simulink library "ITKLib"  (R2022b)
settings: Solver=FixedStepDiscrete  StartTime=0.0  StopTime=10.0  FixedStep=0.01  RelTol=1e-3  EnableMultiTasking=on
values from neighbouring files (symbols this model uses):
  Glb_WhlRollgRd_SC = single(0.36)    [init_Global.m]
undefined symbols (not defined in the file or in its folder): docblock, SlDemoSign, SlDemoSign_Positive_SC, TaskTime_100ms_SC, TaskTime_10ms_SC, VehRefSpd_vMaxRefSpd_C
libraries: simulink x51, $bdroot x45, ITKLib_V14 x1
(part 9 of 10)

== system ITKLib/TimeCounter/CounterRStep ==
  E : Inport  OutDataTypeStr=boolean
  R : Inport  Port=2  OutDataTypeStr=boolean
  Inc : Inport  Port=3
  Constant3 : Constant  Value=Cnt_Max  OutDataTypeStr=uint16  SampleTime=-1
  Limit : Subsystem  Description=""  mask(LIMIT_SL){}
      mask help:
      | GAC Library for Function Development
      |
      | Limits the input value u between the maximum (MX) and the minimum (MN) values.
      |
      | The input value u is checked first against the minimum value and then against the maximum value.
      |
      | In addition to that a flag is set in case the current value is higher than MX and another flag is set in case the current value is smaller than the MN value.
      |
      | inputs:
      | MX  - maximum allowed value
      | MN  - minimal allowed value
      | u   - input value to be evaluated
      |
      | outputs:
      | y       - limited output value
      mask Display:
      | color('black');
      | plot([0.2,0.8],[0.5,0.5]);
      | plot([0.5,0.5],[0.2,0.8]);
      | plot([0.75,0.8,0.75],[0.53,0.5,0.47]);
      | plot([0.53,0.5,0.47],[0.75,0.8,0.75]);
      | color('blue');
      | plot([0.2,0.3,0.7,0.8],[0.3,0.3,0.7,0.7]);
  Limit1 : Subsystem  Description=""  mask(LimitWoFlag){}
      mask help:
      | Limits the input value u between the maximum (MX) and the minimum (MN) values.
      |
      | The input value u is checked first against the minimum value and then against the maximum value.
      |
      | In addition to that a flag is set in case the current value is higher than MX and another flag is set in case the current value is smaller than the MN value.
      |
      | inputs:
      | MX  - maximum allowed value
      | MN  - minimal allowed value
      | u   - input value to be evaluated
      |
      | outputs:
      | y       - limited output value
      |
      | Simulink Custom Model Library, created by MCC.
      mask Display:
      | color('black');
      | plot([0.2,0.8],[0.5,0.5]);
      | plot([0.5,0.5],[0.2,0.8]);
      | plot([0.75,0.8,0.75],[0.53,0.5,0.47]);
      | plot([0.53,0.5,0.47],[0.75,0.8,0.75]);
      | color('blue');
      | plot([0.2,0.3,0.7,0.8],[0.3,0.3,0.7,0.7]);
  Number1 : Constant  Value=65535  OutDataTypeStr=uint16
      settings: AttributesFormatString=%<OutDataTypeStr>
  Number2 : Constant  Value=0  OutDataTypeStr=uint16
      settings: AttributesFormatString=%<OutDataTypeStr>
  Number3 : Constant  Value=0  OutDataTypeStr=uint16
      settings: AttributesFormatString=%<OutDataTypeStr>
  Number8 : Constant  Value=0  OutDataTypeStr=uint16
      settings: AttributesFormatString=%<OutDataTypeStr>
  Saturation2 : Saturate  UpperLimit=uint16(65534)  LowerLimit=uint16(0)
      settings: AttributesFormatString=|
      | UpperLimit = %<UpperLimit>
      | LowLimit = %<LowerLimit>
  Sum : Sum  InputSameDT=on  OutDataTypeStr=uint16  SaturateOnIntegerOverflow=on
  Switch1 : Switch  Criteria=u2 ~= 0  OutDataTypeStr=uint16
      settings: AttributesFormatString=threshold=%<threshold>\nCriteria : %<Criteria>
  Switch2 : Switch  Criteria=u2 ~= 0
      settings: AttributesFormatString=threshold=%<threshold>\nCriteria : %<Criteria>
  Unit Delay1 : UnitDelay  InitialCondition=uint16(0)  SampleTime=-1  HasFrameUpgradeWarning=on
      settings: AttributesFormatString=<initial=%<x0>>
  Cnt : Outport
  wires:
  E/1 -> Switch1/2
  Unit Delay1/1 -> Sum/2, Switch1/3
  Number2/1 -> Switch2/1
  Sum/1 -> Saturation2/1
  Switch1/1 -> Switch2/3
  Inc/1 -> Limit/2(u)
  R/1 -> Switch2/2
  Limit1/1(y) -> Cnt/1, Unit Delay1/1
  Switch2/1 -> Limit1/2(u)
  Constant3/1 -> Limit1/1(MX)
  Number3/1 -> Limit1/3(MN)
  Limit/1(y) -> Sum/1
  Number1/1 -> Limit/1(MX)
  Number8/1 -> Limit/3(MN)
  Saturation2/1 -> Switch1/1

== system ITKLib/TimeCounter/DebCnt ==
  bErr : Inport  OutDataTypeStr=boolean
  bRst : Inport  Port=2  OutDataTypeStr=boolean
  bEna : Inport  Port=3  OutDataTypeStr=boolean  PortDimensions=1
  FailThd : Inport  Port=4  OutDataTypeStr=int16
  RcvThd : Inport  Port=5  OutDataTypeStr=int16
  IncFail : Inport  Port=6  OutDataTypeStr=int16
  DecRcv : Inport  Port=7  OutDataTypeStr=int16
  DebounceEnable : Subsystem
  Debounce_OBD : Subsystem  TreatAsAtomicUnit=on
  Unit Delay1 : UnitDelay  SampleTime=-1  HasFrameUpgradeWarning=on
      settings: AttributesFormatString=<initial=%<X0>>
  Unit Delay2 : UnitDelay  SampleTime=-1  HasFrameUpgradeWarning=on
      settings: AttributesFormatString=<initial=%<X0>>
  bFaild : Outport
  wires:
  DecRcv/1 -> Debounce_OBD/6(DecrRec)
  IncFail/1 -> Debounce_OBD/5(IncrFail)
  Debounce_OBD/2(bFaild) -> Unit Delay1/1, bFaild/1
  bErr/1 -> DebounceEnable/5(bErr), Debounce_OBD/1(bErr)
  bRst/1 -> Debounce_OBD/2(bRst), DebounceEnable/4(bRst)
  FailThd/1 -> Debounce_OBD/3(FailThd)
  RcvThd/1 -> Debounce_OBD/4(RecThd)
  bEna/1 -> DebounceEnable/3(bEna)
  Debounce_OBD/1(bOutRanged) -> Unit Delay2/1
  DebounceEnable/1(bDebounceEna) -> Debounce_OBD/Enable
  Unit Delay2/1 -> DebounceEnable/1(bOutRangedOld)
  Unit Delay1/1 -> DebounceEnable/2(bFailedOld)

== system ITKLib/TimeCounter/Debounce ==
  In : Inport  OutDataTypeStr=boolean
  R : Inport  Port=2
  TAct : Inport  Port=3
  TDeact : Inport  Port=4
  dT : Inport  Port=5
  Constant2 : Constant  Value=IV  OutDataTypeStr=boolean  SampleTime=-1
  Logical Operator1 : Logic  Operator=NOT  AllPortsSameDT=off  OutDataTypeStr=boolean
  OR : Logic  Operator=OR  OutDataTypeStr=boolean
  RSLatchIV : Subsystem  RTWFcnName=RS_Latch_IV_Pos  RTWFileName=SEN_MDL_LIB  mask(RSLatchIV){}
      mask help:
      | RS latch with initial value
      | Set signal is passed from port 'S'
      | Reset signal is passed from port 'R'
      | Initial value is passed from port 'IV'
      |
      | Q is set if S is set and reset if R is set.
      | The reset logic is of higher priority than set logic.
      | The initial state is set by IV.
      |
      | Simulink Custom Model Library, created by MCC.
      settings: MinAlgLoopOccurrences=on  RTWFcnNameOpts=User specified  RTWFileNameOpts=User specified
      mask Help:
      | RS latch with initial value
      | Set signal is passed from port 'S'
      | Reset signal is passed from port 'R'
      | Initial value is passed from port 'IV'
      | 
      | Q is set if S is set and reset if R is set.
      | The reset logic is of higher priority than set logic.
      | The initial state is set by IV.
      mask Display:
      | color('blue')
      | disp('\fontsize{12}RS Latch', 'texmode', 'on')
      | color('black');
      | port_label('input', 1, 'S', 'texmode', 'on')
      | port_label('input', 2, 'R', 'texmode', 'on')
      | port_label('input', 3, 'IV', 'texmode', 'on')
      | port_label('output', 1, 'Q', 'texmode', 'on')
      | %text(1,0,'SEN','horizontalAlignment','right','verticalAlignment','bottom');
  TurnOnDelayVari : $bdroot/TimeCounter/TurnOnDelayVari
      settings: AttributesFormatString=TurnOnDelay
  TurnOnDelayVari1 : $bdroot/TimeCounter/TurnOnDelayVari
      settings: AttributesFormatString=TurnOnDelay
  Out : Outport  OutDataTypeStr=boolean
  wires:
  Constant2/1 -> RSLatchIV/3(IV)
  RSLatchIV/1(Q) -> Out/1
  TAct/1 -> TurnOnDelayVari/3
  dT/1 -> [dT], TurnOnDelayVari/2
  TDeact/1 -> TurnOnDelayVari1/3
  In/1 -> TurnOnDelayVari/1, Logical Operator1/1
  Logical Operator1/1 -> TurnOnDelayVari1/1
  TurnOnDelayVari/1 -> RSLatchIV/1(S)
  R/1 -> OR/2
  OR/1 -> RSLatchIV/2(R)
  TurnOnDelayVari1/1 -> OR/1
  [dT] -> TurnOnDelayVari1/2

== system ITKLib/TimeCounter/StopWatchRE ==
  E : Inport  OutDataTypeStr=boolean
  R : Inport  Port=2  OutDataTypeStr=boolean
  dT : Inport  Port=3
  Number1 : Constant  Value=0  OutDataTypeStr=single
      settings: AttributesFormatString=%<OutDataTypeStr>
  Sum1 : Sum  SaturateOnIntegerOverflow=on
  Switch1 : Switch  Criteria=u2 ~= 0  SaturateOnIntegerOverflow=off  InputSameDT=off
      settings: AttributesFormatString=Criteria : %<Criteria>
  Switch2 : Switch  Criteria=u2 ~= 0  SaturateOnIntegerOverflow=off  InputSameDT=off
      settings: AttributesFormatString=Criteria : %<Criteria>
  Unit Delay1 : UnitDelay  SampleTime=-1  HasFrameUpgradeWarning=on
      settings: AttributesFormatString=<initial=%<x0>>
  y : Outport
  wires:
  dT/1 -> Sum1/1
  Switch2/1 -> y/1, Unit Delay1/1
  Switch1/1 -> Switch2/3
  E/1 -> Switch1/2
  Number1/1 -> Switch2/1
  R/1 -> Switch2/2
  Unit Delay1/1 -> Switch1/3, Sum1/2
  Sum1/1 -> Switch1/1

== system ITKLib/TimeCounter/TurnOnDelayVari ==
  In : Inport  OutDataTypeStr=boolean
  dT : Inport  Port=2
  T : Inport  Port=3
  DataTypeConversion : DataTypeConversion  OutDataTypeStr=int32  RndMeth=Nearest  SaturateOnIntegerOverflow=off
  Divide : Product  Inputs=*/  InputSameDT=on  SaturateOnIntegerOverflow=on
  Max : MinMax  Function=max  Inputs=2  InputSameDT=on  SaturateOnIntegerOverflow=on
  Relational Operator1 : RelationalOperator  Operator=>  OutDataTypeStr=boolean
  Saturation2 : Saturate  UpperLimit=2147483647  LowerLimit=-2147483648
      settings: AttributesFormatString=|
      | UpperLimit = %<UpperLimit>
      | LowLimit = %<LowerLimit>
  Subtract1 : Sum  InputSameDT=on  SaturateOnIntegerOverflow=on
  Switch : Switch  Criteria=u2 ~= 0  SaturateOnIntegerOverflow=off  InputSameDT=off
      settings: AttributesFormatString=Criteria : %<Criteria>
  Unit Delay : UnitDelay  InitialCondition=int32(0)  SampleTime=-1  HasFrameUpgradeWarning=on
      settings: AttributesFormatString=<initial=%<x0>>
  single1 : Constant  OutDataTypeStr=int32
      settings: AttributesFormatString=%<OutDataTypeStr>
  single2 : Constant  Value=0  OutDataTypeStr=int32
      settings: AttributesFormatString=%<OutDataTypeStr>
  single3 : Constant  Value=0.0001  OutDataTypeStr=single
      settings: AttributesFormatString=%<OutDataTypeStr>
  Out : Outport  OutDataTypeStr=boolean
  wires:
  single2/1 -> Switch/3
  In/1 -> Switch/2
  Switch/1 -> Saturation2/1
  Relational Operator1/1 -> Out/1
  Subtract1/1 -> Switch/1
  Unit Delay/1 -> Subtract1/1
  single1/1 -> Subtract1/2
  Divide/1 -> DataTypeConversion/1
  DataTypeConversion/1 -> Relational Operator1/2
  T/1 -> Divide/1
  dT/1 -> Max/1
  single3/1 -> Max/2
  Max/1 -> Divide/2
  Saturation2/1 -> Unit Delay/1, Relational Operator1/1

== system ITKLib/TimeCounter/Turn_Off_Delay_Vari ==
  In : Inport  OutDataTypeStr=boolean
  dT : Inport  Port=2
  T : Inport  Port=3
  DataTypeConversion : DataTypeConversion  OutDataTypeStr=int32  RndMeth=Nearest  SaturateOnIntegerOverflow=off
  Divide : Product  Inputs=*/  InputSameDT=on  SaturateOnIntegerOverflow=on
  Logical Operator2 : Logic  Operator=OR  AllPortsSameDT=off  OutDataTypeStr=boolean
  Max : MinMax  Function=max  Inputs=2  InputSameDT=on  SaturateOnIntegerOverflow=on
  Relational Operator : RelationalOperator  Operator=>  OutDataTypeStr=boolean  InputSameDT=off
  Saturation2 : Saturate  UpperLimit=2147483647  LowerLimit=-2147483648
      settings: AttributesFormatString=|
      | UpperLimit = %<UpperLimit>
      | LowLimit = %<LowerLimit>
  Subtract : Sum  Inputs=+-
  Switch : Switch  Criteria=u2 ~= 0  SaturateOnIntegerOverflow=off  InputSameDT=off
      settings: AttributesFormatString=Criteria : %<Criteria>
  Switch1 : Switch  Criteria=u2 ~= 0  SaturateOnIntegerOverflow=off  InputSameDT=off
      settings: AttributesFormatString=Criteria : %<Criteria>
  Unit Delay : UnitDelay  InitialCondition=uint32(0)  SampleTime=-1  HasFrameUpgradeWarning=on
      settings: AttributesFormatString=<initial=%<x0>>
  single3 : Constant  Value=0.0001  OutDataTypeStr=single
      settings: AttributesFormatString=%<OutDataTypeStr>
  single4 : Constant  Value=0  OutDataTypeStr=int32
      settings: AttributesFormatString=%<OutDataTypeStr>
  single5 : Constant  OutDataTypeStr=int32
      settings: AttributesFormatString=%<OutDataTypeStr>
  Out : Outport  OutDataTypeStr=boolean
  wires:
  Switch/1 -> Saturation2/1
  single4/1 -> Relational Operator/2
  Logical Operator2/1 -> Out/1
  Switch1/1 -> Switch/3
  Relational Operator/1 -> Switch1/2, [TimeFlag]
  In/1 -> Switch/2, Logical Operator2/2
  Unit Delay/1 -> Subtract/1, Relational Operator/1, Switch1/3
  Subtract/1 -> Switch1/1
  [TimeFlag] -> Logical Operator2/1
  DataTypeConversion/1 -> Switch/1
  single5/1 -> Subtract/2
  Max/1 -> Divide/2
  single3/1 -> Max/2
  dT/1 -> Max/1
  T/1 -> Divide/1
  Divide/1 -> DataTypeConversion/1
  Saturation2/1 -> Unit Delay/1

== system ITKLib/BasicOperators/Drvt/MaxITK ==
  In1 : Inport
  In2 : Inport  Port=2
  Greater : RelationalOperator  Operator=>  OutDataTypeStr=boolean
  Switch : Switch  Criteria=u2 ~= 0  SaturateOnIntegerOverflow=off  InputSameDT=off
      settings: AttributesFormatString=Criteria : %<Criteria>
  Out1 : Outport  VectorParamsAs1DForOutWhenUnconnected=off
  wires:
  In1/1 -> Switch/1, Greater/1
  In2/1 -> Switch/3, Greater/2
  Greater/1 -> Switch/2
  Switch/1 -> Out1/1

== system ITKLib/BasicOperators/Int32ToSingle/Opposite ==
  In : Inport
  Product2 : Product  InputSameDT=on  SaturateOnIntegerOverflow=on
  single : Constant  Value=-1  OutDataTypeStr=single
      settings: AttributesFormatString=%<OutDataTypeStr>
  " Out " : Outport
  wires:
  single/1 -> Product2/2
  Product2/1 -> " Out "/1
  In/1 -> Product2/1

== system ITKLib/BasicOperators/Safe_Divide/Opposite ==
  In : Inport
  Product2 : Product  InputSameDT=on  SaturateOnIntegerOverflow=on
  single : Constant  Value=-1  OutDataTypeStr=single
      settings: AttributesFormatString=%<OutDataTypeStr>
  " Out " : Outport
  wires:
  single/1 -> Product2/2
  Product2/1 -> " Out "/1
  In/1 -> Product2/1

== system ITKLib/BasicOperators/Safe_Divide/Opposite1 ==
  In : Inport
  Product2 : Product  InputSameDT=on  SaturateOnIntegerOverflow=on
  single : Constant  Value=-1  OutDataTypeStr=single
      settings: AttributesFormatString=%<OutDataTypeStr>
  " Out " : Outport
  wires:
  single/1 -> Product2/2
  Product2/1 -> " Out "/1
  In/1 -> Product2/1

== system ITKLib/Diagnosis/Debounce_OBD/DebounceEnable ==
  bOutRangedOld : Inport
  bFailedOld : Inport  Port=2
  bEna : Inport  Port=3  OutDataTypeStr=boolean  PortDimensions=1
  bRst : Inport  Port=4
  bErr : Inport  Port=5
  Logical Operator : Logic  Operator=OR  OutDataTypeStr=boolean
  Logical Operator1 : Logic  OutDataTypeStr=boolean
  Logical Operator2 : Logic  Operator=NOT  Inputs=1  AllPortsSameDT=off  OutDataTypeStr=boolean
  Logical Operator3 : Logic  OutDataTypeStr=boolean
  Logical Operator4 : Logic  Inputs=1  AllPortsSameDT=off  OutDataTypeStr=boolean
  Relational Operator : RelationalOperator  Operator===  OutDataTypeStr=boolean
  bDebounceEna : Outport
  wires:
  bEna/1 -> Logical Operator3/2
  Logical Operator3/1 -> Logical Operator/1
  Logical Operator/1 -> bDebounceEna/1
  Relational Operator/1 -> Logical Operator1/2
  Logical Operator1/1 -> Logical Operator4/1
  Logical Operator2/1 -> Logical Operator3/1
  bOutRangedOld/1 -> Logical Operator1/1
  Logical Operator4/1 -> Logical Operator2/1
  bErr/1 -> Relational Operator/2
  bRst/1 -> Logical Operator/2
  bFailedOld/1 -> Relational Operator/1

== system ITKLib/Diagnosis/Debounce_OBD/Debounce_OBD ==
  note: test run failure always causes fault detection counter to increment above 0
      | (so as not to double the fail detection time following a test complete with pass)
  note: only if the FaultDetectionCounter less than 0
  note: rising edge detection
  note: FailCtr <= errCtr <= RecoverCtr
  bErr : Inport
  bRst : Inport  Port=2
  FailThd : Inport  Port=3
  RecThd : Inport  Port=4
  IncrFail : Inport  Port=5
  DecrRec : Inport  Port=6
  Enable : EnablePort
  EdgeRising : $bdroot/Memory/EdgeRising  Tag=initial value = 0
  LORelay1 : Logic  Operator=OR  AllPortsSameDT=off  OutDataTypeStr=boolean
  Logical Operator : Logic  OutDataTypeStr=boolean
  ROLoLim : RelationalOperator  Operator=<  OutDataTypeStr=boolean  InputSameDT=off
  ROUpLim : RelationalOperator  Operator=<  OutDataTypeStr=boolean  InputSameDT=off
  RSLatch : $bdroot/Memory/RSLatch
  Relational Operator : RelationalOperator  Operator=<  OutDataTypeStr=boolean
  Saturation2 : Saturate  UpperLimit=int16(32766)  LowerLimit=int16(-32767)
      settings: AttributesFormatString=|
      | UpperLimit = %<UpperLimit>
      | LowLimit = %<LowerLimit>
  Sum1 : Sum  InputSameDT=on  OutDataTypeStr=int16  SaturateOnIntegerOverflow=on
  Sum2 : Sum  InputSameDT=on  OutDataTypeStr=int16  SaturateOnIntegerOverflow=on
  Switch{,2..4} (4 alike) : Switch  Criteria=u2 ~= 0  SaturateOnIntegerOverflow=off  InputSameDT=off
      settings: AttributesFormatString=Criteria : %<Criteria>
  Unit Delay : UnitDelay  SampleTime=-1  HasFrameUpgradeWarning=on
      settings: AttributesFormatString=<initial=%<X0>>
  int1 : Constant  Value=0  OutDataTypeStr=int16
      settings: AttributesFormatString=%<OutDataTypeStr>
  int16 : Constant  Value=0  OutDataTypeStr=int16
      settings: AttributesFormatString=%<OutDataTypeStr>
  bOutRanged : Outport  InitialOutput=0
  bFailed : Outport  Port=2  InitialOutput=0
  wires:
  [bRst] -> Switch2/2
  Switch2/1 -> Switch3/1, Sum2/2, Sum1/2
  Switch/1 -> Switch2/3
  int16/1 -> Switch2/1, Switch/1
  RSLatch/1 -> bFailed/1
  Sum1/1 -> Switch4/1
  Sum2/1 -> Switch4/3
  Switch3/1 -> Unit Delay/1
  DecrRec/1 -> Sum2/1
  IncrFail/1 -> Sum1/1
  bErr/1 -> Switch4/2, EdgeRising/1
  Logical Operator/1 -> Switch/2
  Relational Operator/1 -> Logical Operator/2
  int1/1 -> Relational Operator/2
  EdgeRising/1 -> Logical Operator/1
  Unit Delay/1 -> Relational Operator/1, Switch/3
  bRst/1 -> [bRst], LORelay1/2
  RecThd/1 -> ROLoLim/2
  ROUpLim/1 -> RSLatch/1, Switch3/2, bOutRanged/1  "outRanged"
  Switch4/1 -> Saturation2/1
  ROLoLim/1 -> LORelay1/1
  FailThd/1 -> ROUpLim/1
  LORelay1/1 -> RSLatch/2
  Saturation2/1 -> Switch3/3, ROLoLim/1, ROUpLim/2

== system ITKLib/Diagnosis/FltCollctn/FltPos ==
  FltNr : Inport
  Divide : Product  Inputs=*/
  Math Function : Math  Operator=mod  SignedPower=on
  uint8 : Constant  Value=16  OutDataTypeStr=uint8  SampleTime=-1
      settings: AttributesFormatString=%<OutDataTypeStr>
  AryIdx : Outport
  BitPos : Outport  Port=2
  wires:
  Math Function/1 -> BitPos/1
  Divide/1 -> AryIdx/1
  FltNr/1 -> Divide/1, Math Function/1
  uint8/1 -> Math Function/2, Divide/2

== system ITKLib/Diagnosis/FltLatchCollctn/FltPos ==
  FltNr : Inport
  Divide : Product  Inputs=*/
  Math Function : Math  Operator=mod  SignedPower=on
  uint8 : Constant  Value=16  OutDataTypeStr=uint8  SampleTime=-1
      settings: AttributesFormatString=%<OutDataTypeStr>
  AryIdx : Outport
  BitPos : Outport  Port=2
  wires:
  uint8/1 -> Divide/2, Math Function/2
  FltNr/1 -> Math Function/1, Divide/1
  Divide/1 -> AryIdx/1
  Math Function/1 -> BitPos/1

== system ITKLib/Diagnosis/FltLatchCollctn/Subsystem ==
  FltNr : Inport
  FltFlg : Inport  Port=2
  SentCod : Inport  Port=3
  AND : Logic  OutDataTypeStr=boolean
  Demux : Demux
  Equal{,1..3} (4 alike) : RelationalOperator  Operator===  OutDataTypeStr=boolean  RndMeth=Simplest  InputSameDT=off
  Not : Logic  Operator=NOT  AllPortsSameDT=off  OutDataTypeStr=boolean
  OR : Logic  Operator=OR  Inputs=4  OutDataTypeStr=boolean
  RSLatch : $bdroot/Memory/RSLatch
  FltFlg1 : Outport
  wires:
  FltFlg/1 -> Not/1, RSLatch/1
  Demux/1 -> Equal/1
  Not/1 -> AND/2
  Demux/4 -> Equal3/1
  AND/1 -> RSLatch/2
  FltNr/1 -> Equal/2, Equal1/2, Equal2/2, Equal3/2
  Equal2/1 -> OR/3
  Demux/2 -> Equal1/1
  Equal3/1 -> OR/4
  Equal/1 -> OR/1
  OR/1 -> AND/1
  Equal1/1 -> OR/2
  Demux/3 -> Equal2/1
  RSLatch/1 -> FltFlg1/1
  SentCod/1 -> Demux/1

== system ITKLib/Diagnosis/RollgCntrChk/RSLatch ==
  S : Inport  OutDataTypeStr=boolean
  R : Inport  Port=2  OutDataTypeStr=boolean
  Logical Operator1 : Logic  Operator=NOT  AllPortsSameDT=off  OutDataTypeStr=boolean
  Logical_Operator4 : Logic  AllPortsSameDT=off  OutDataTypeStr=boolean
  Logical_Operator5 : Logic  Operator=OR  AllPortsSameDT=off  OutDataTypeStr=boolean
  Unit Delay : UnitDelay  SampleTime=-1  HasFrameUpgradeWarning=on
      settings: AttributesFormatString=<initial=%<x0>>
  Q : Outport  OutDataTypeStr=boolean
  wires:
  Unit Delay/1 -> Logical_Operator5/2
  Logical_Operator4/1 -> Q/1, Unit Delay/1
  Logical Operator1/1 -> Logical_Operator4/1
  Logical_Operator5/1 -> Logical_Operator4/2
  R/1 -> Logical Operator1/1
  S/1 -> Logical_Operator5/1

== system ITKLib/Filter/MoveAvrgFilt/Limit1 ==
  MX : Inport
  u : Inport  Port=2
  MN : Inport  Port=3
  GreaterOrEqual : RelationalOperator  OutDataTypeStr=boolean
  MinMax : MinMax  Inputs=2  SaturateOnIntegerOverflow=on
  MinMax1 : MinMax  Function=max  Inputs=2  SaturateOnIntegerOverflow=on
  MinMax2 : MinMax  Function=max  Inputs=2  SaturateOnIntegerOverflow=on
  MinMax3 : MinMax  Inputs=2  SaturateOnIntegerOverflow=on
  Switch : Switch  Criteria=u2 ~= 0  SaturateOnIntegerOverflow=off  InputSameDT=off
      settings: AttributesFormatString=Criteria : %<Criteria>
  y : Outport  InitialOutput=0
  wires:
  [MX] -> MinMax/1
  [MN] -> MinMax1/2
  MinMax3/1 -> Switch/3
  [MN] -> MinMax3/2
  MinMax2/1 -> MinMax3/1
  [MX] -> MinMax2/2
  [u] -> MinMax2/1
  MinMax/1 -> Switch/1
  GreaterOrEqual/1 -> Switch/2
  Switch/1 -> y/1
  MinMax1/1 -> MinMax/2
  MN/1 -> GreaterOrEqual/2, [MN]
  u/1 -> MinMax1/1, [u]
  MX/1 -> GreaterOrEqual/1, [MX]

== system ITKLib/Filter/SecOrdBPF/DisableFilterDeal ==
  Input : Inport
  ActionPort : ActionPort  InitializeStates=reset  ActionPortLabel=else
  Output : Outport
  wires:
  Input/1 -> Output/1

== system ITKLib/Filter/SecOrdBPF/FilterJudgment ==
  FilterTime : Inport
  SampleTime : Inport  Port=2
  LogicalOperator : Logic  AllPortsSameDT=off  OutDataTypeStr=boolean
  RelationalOperator : RelationalOperator  Operator=>  OutDataTypeStr=boolean  RndMeth=Simplest  InputSameDT=off
  RelationalOperator2 : RelationalOperator  Operator=>  OutDataTypeStr=boolean  RndMeth=Simplest  InputSameDT=off
  single4 : Constant  Value=0  OutDataTypeStr=single  SampleTime=-1
      settings: AttributesFormatString=%<OutDataTypeStr>
  u1 : Outport
  wires:
  LogicalOperator/1 -> u1/1
  RelationalOperator2/1 -> LogicalOperator/2
  single4/1 -> RelationalOperator2/2
  RelationalOperator/1 -> LogicalOperator/1
  SampleTime/1 -> RelationalOperator/2, RelationalOperator2/1
  FilterTime/1 -> RelationalOperator/1

== system ITKLib/Filter/SecOrdBPF/If Action Subsystem ==
  in : Inport
  FltOutOld : Inport  Port=2
  Omega : Inport  Port=3
  Zeta : Inport  Port=4
  SmpTime : Inport  Port=5
  Action Port : ActionPort  InitializeStates=reset  ActionPortLabel=if(u1 ~=0)
  Add : Sum  Inputs=+++
  Add1 : Sum  Inputs=+-+
  Add2 : Sum  Inputs=+-
  Add3 : Sum  Inputs=+---
  Delay : Delay
  Divide : Product  Inputs=*/  OutDataTypeStr=single  RndMeth=Simplest
      settings: AttributesFormatString=RndMeth=%<RndMeth>
  Dot Product : DotProduct  OutDataTypeStr=Inherit: Inherit via internal rule
  Dot Product1 : DotProduct  OutDataTypeStr=Inherit: Inherit via internal rule
  Product : Product  Inputs=4
  Product{1..6} (6 alike) : Product
  Unit Delay1 : UnitDelay  SampleTime=-1  HasFrameUpgradeWarning=on
  single1 : Constant  Value=2  OutDataTypeStr=single  SampleTime=-1
      settings: AttributesFormatString=%<OutDataTypeStr>
  single2 : Constant  Value=8  OutDataTypeStr=single  SampleTime=-1
      settings: AttributesFormatString=%<OutDataTypeStr>
  single4 : Constant  Value=4  OutDataTypeStr=single  SampleTime=-1
      settings: AttributesFormatString=%<OutDataTypeStr>
  FltOut : Outport
  wires:
  [d] -> Product6/2
  [e] -> Product5/2
  Product6/1 -> Add3/4
  Product5/1 -> Add3/3
  [a] -> Product4/2
  Product4/1 -> Add3/1
  [b] -> Product3/2
  Product3/1 -> Add3/2
  Delay/1 -> Product3/1  "u(k-2)"
  Unit Delay1/1 -> Product5/1  "Y(k-2)"
  FltOutOld/1 -> Unit Delay1/1, Product6/1  "Y(k-1)"
  in/1 -> Delay/1, Product4/1
  Add3/1 -> Divide/1
  [c] -> Divide/2
  Add2/1 -> [d]
  single2/1 -> Add2/2
  single1/1 -> Product1/2
  Product1/1 -> Add2/1
  Add1/1 -> [e]
  Add/1 -> [c]
  Product2/1 -> Add1/3, Product1/1, Add/3
  Dot Product/1 -> Product2/1
  Dot Product1/1 -> Product2/2
  Product/1 -> [b], Add/1, Add1/2, [a]
  Omega/1 -> Dot Product/2, Dot Product/1, Product/2
  Zeta/1 -> Product/3
  SmpTime/1 -> Product/4, Dot Product1/1, Dot Product1/2
  single4/1 -> Product/1, Add/2, Add1/1
  Divide/1 -> FltOut/1

== system ITKLib/PID/PIGovernor/I ==
  u : Inport
  PreC : Inport  Port=2
  Max : Inport  Port=3
  Min : Inport  Port=4
  Ki : Inport  Port=5
  Ena : Inport  Port=6  OutDataTypeStr=boolean
  R : Inport  Port=7  OutDataTypeStr=boolean
  RV : Inport  Port=8
  dT : Inport  Port=9
  Add : Sum  InputSameDT=on  SaturateOnIntegerOverflow=on
  Greater : RelationalOperator  Operator=>  OutDataTypeStr=boolean
  Lower : RelationalOperator  Operator=<  OutDataTypeStr=boolean
  Max1 : MinMax  Function=max  Inputs=2  InputSameDT=on  SaturateOnIntegerOverflow=on
  Max3 : MinMax  Function=max  Inputs=2  InputSameDT=on  SaturateOnIntegerOverflow=on
  Min1 : MinMax  Inputs=2  InputSameDT=on  SaturateOnIntegerOverflow=on
  Min3 : MinMax  Inputs=2  InputSameDT=on  SaturateOnIntegerOverflow=on
  Product : Product  InputSameDT=on  SaturateOnIntegerOverflow=on
  Product1 : Product  InputSameDT=on  SaturateOnIntegerOverflow=on
  Subtract : Sum  Inputs=+-  InputSameDT=on  SaturateOnIntegerOverflow=on
  Subtract1 : Sum  Inputs=+-  InputSameDT=on  SaturateOnIntegerOverflow=on
  Switch{1..4} (4 alike) : Switch  Criteria=u2 ~= 0  SaturateOnIntegerOverflow=off  InputSameDT=off
      settings: AttributesFormatString=Criteria : %<Criteria>
  Unit Delay1 : UnitDelay  SampleTime=-1  HasFrameUpgradeWarning=on
      settings: AttributesFormatString=<initial=%<x0>>
  UnitDelay : UnitDelay  SampleTime=-1  HasFrameUpgradeWarning=on
      settings: AttributesFormatString=<Initial=%<x0>>
  UnitDelay1 : UnitDelay  SampleTime=-1  HasFrameUpgradeWarning=on
      settings: AttributesFormatString=<Initial=%<x0>>
  uint3 : Constant  Value=0  OutDataTypeStr=single
  uint4 : Constant  Value=0  OutDataTypeStr=single
  KiOut : Outport
  wires:
  [StepHiLmt] -> UnitDelay1/1
  Max1/1 -> Switch1/1
  UnitDelay1/1 -> Switch4/2
  Switch2/1 -> Switch3/3
  Switch3/1 -> [yRaw], Max3/2
  Switch4/1 -> Add/1
  Add/1 -> Switch2/1
  Ena/1 -> Switch2/2
  R/1 -> Switch3/2
  Unit Delay1/1 -> Switch2/3, Add/2
  Product/1 -> Product1/1
  PreC/1 -> Subtract1/2, Subtract/2
  uint4/1 -> Max1/2
  Lower/1 -> [StepHiLmt]
  Max3/1 -> Min3/2
  RV/1 -> Switch3/1
  Ki/1 -> Product/2
  Subtract1/1 -> Min3/1
  Greater/1 -> [StepLoLmt]
  [yRaw] -> Greater/2
  Switch1/1 -> Switch4/3
  u/1 -> Product/1
  Min1/1 -> Switch4/1
  Subtract/1 -> Max3/1
  UnitDelay/1 -> Switch1/2
  Max/1 -> Subtract1/1
  uint3/1 -> Min1/2
  Min/1 -> Subtract/1
  [StepLoLmt] -> UnitDelay/1
  dT/1 -> Product1/2
  Product1/1 -> Switch1/3, Max1/1, Min1/1
  [yRaw] -> Lower/2
  Min3/1 -> Greater/1, Unit Delay1/1, Lower/1, KiOut/1

== system ITKLib/PID/PIGovernor/P ==
  u : Inport
  Kp : Inport  Port=2
  Product : Product  RndMeth=Zero
  KpOut : Outport
  wires:
  Product/1 -> KpOut/1
  u/1 -> Product/1
  Kp/1 -> Product/2

== system ITKLib/PID/PIGovernor/PILim ==
  Prec : Inport
  KpOut : Inport  Port=2
  KiOut : Inport  Port=3
  Min : Inport  Port=4
  Max : Inport  Port=5
  Ena : Inport  Port=6
  Add : Sum  Inputs=+++
  Max1 : MinMax  Function=max  Inputs=2  InputSameDT=on  SaturateOnIntegerOverflow=on
  Min1 : MinMax  Inputs=2  InputSameDT=on  SaturateOnIntegerOverflow=on
  Switch2 : Switch  Criteria=u2 ~= 0  SaturateOnIntegerOverflow=off  InputSameDT=off
      settings: AttributesFormatString=Criteria : %<Criteria>
  Unit Delay1 : UnitDelay  SampleTime=-1  HasFrameUpgradeWarning=on
      settings: AttributesFormatString=<initial=%<x0>>
  PIOut : Outport
  wires:
  KpOut/1 -> Add/2
  Prec/1 -> Add/1
  KiOut/1 -> Add/3
  Switch2/1 -> PIOut/1, Unit Delay1/1
  Min1/1 -> Switch2/1
  Max1/1 -> Min1/2
  Min/1 -> Max1/1
  Ena/1 -> Switch2/2
  Add/1 -> Max1/2
  Max/1 -> Min1/1
  Unit Delay1/1 -> Switch2/3

== system ITKLib/Special/ControlAlgorithm/AdrcCtrl ==
  yTar : Inport
  y : Inport  Port=2
  r : Inport  Port=3
  h : Inport  Port=4
  Ts : Inport  Port=5
  DlyCnt : Inport  Port=6
  ESO_Alpha1 : Inport  Port=7
  ESO_Beta1 : Inport  Port=8
  ESO_Dlt : Inport  Port=9
  ESO_Alpha2 : Inport  Port=10
  ESO_Beta2 : Inport  Port=11
  ESO_Alpha3 : Inport  Port=12
  ESO_Beta3 : Inport  Port=13
  b : Inport  Port=14
  NLSEF_Alpha0 : Inport  Port=15
  NLSEF_Beta0 : Inport  Port=16
  NLSEF_Alpha1 : Inport  Port=17
  NLSEF_Beta1 : Inport  Port=18
  NLSEF_Dlt : Inport  Port=19
  NLSEF_Alpha2 : Inport  Port=20
  NLSEF_Beta2 : Inport  Port=21
  dT : Inport  Port=22
  CalcActDrvt : Subsystem
  ESO : Subsystem
  NLSEF : Subsystem
  TD : Subsystem
  UnitDelay : UnitDelay  SampleTime=-1  HasFrameUpgradeWarning=on
      settings: AttributesFormatString=<Initial=%<x0>>
  u : Outport  VectorParamsAs1DForOutWhenUnconnected=off
  wires:
  TD/2(z12) -> NLSEF/2(z12)
  NLSEF/1(u) -> u/1, UnitDelay/1
  TD/1(z11) -> NLSEF/1(z11)
  ESO/1(z23) -> NLSEF/5(z23)
  yTar/1 -> TD/1(yd)
  y/1 -> CalcActDrvt/3(y), NLSEF/4(z21), ESO/1(y)
  UnitDelay/1 -> ESO/11(u)
  r/1 -> TD/2(r)
  h/1 -> TD/3(h)
  Ts/1 -> TD/4(Ts)
  CalcActDrvt/1(ActInpDrvt) -> NLSEF/3(z22)
  DlyCnt/1 -> CalcActDrvt/1(DlyCnt)
  dT/1 -> [dT], CalcActDrvt/2(dT)
  [dT] -> ESO/2(dT)
  [dT] -> NLSEF/6(dT)
  ESO_Alpha1/1 -> ESO/3(ESO_Alpha1)
  ESO_Beta1/1 -> ESO/4(ESO_Beta1)
  ESO_Dlt/1 -> ESO/5(ESO_Dlt)
  ESO_Alpha2/1 -> ESO/6(ESO_Alpha2)
  ESO_Beta2/1 -> ESO/7(ESO_Beta2)
  ESO_Alpha3/1 -> ESO/8(ESO_Alpha3)
  ESO_Beta3/1 -> ESO/9(ESO_Beta3)
  b/1 -> [b], ESO/10(b)
  [b] -> NLSEF/7(b)
  NLSEF_Alpha0/1 -> NLSEF/8(NLSEF_Alpha0)
  NLSEF_Beta0/1 -> NLSEF/9(NLSEF_Beta0)
  NLSEF_Alpha1/1 -> NLSEF/10(NLSEF_Alpha1)
  NLSEF_Beta1/1 -> NLSEF/11(NLSEF_Beta1)
  NLSEF_Dlt/1 -> NLSEF/12(NLSEF_Dlt)
  NLSEF_Beta2/1 -> NLSEF/14(NLSEF_Beta2)
  NLSEF_Alpha2/1 -> NLSEF/13(NLSEF_Alpha2)

== system ITKLib/Special/ControlAlgorithm/Lgtd_Lat_Force ==
  VfASR_WhlSlipRat_coff : Inport
  VfDTC_WhlSlipRat_coff : Inport  Port=2
  VfACE_WhlAdhCoff_coff : Inport  Port=3
  VfVME_WhlVertF_N : Inport  Port=4
  VfVDM_TireSideSlipAng_deg : Inport  Port=5
  KfVDM_TireLgtdStfn_Npm : Inport  Port=6
  KfVDM_TireCornrgStfn_Npm : Inport  Port=7
  Add : Sum  Inputs=-+  InputSameDT=on  SaturateOnIntegerOverflow=on
  Add1 : Sum  InputSameDT=on  SaturateOnIntegerOverflow=on
  Add2 : Sum  Inputs=+-  InputSameDT=on  SaturateOnIntegerOverflow=on
  Add3 : Sum  Inputs=-+  InputSameDT=on  SaturateOnIntegerOverflow=on
  Divide : Product  Inputs=*/  InputSameDT=on  RndMeth=Zero  SaturateOnIntegerOverflow=on
  Divide1 : Product  Inputs=***//  InputSameDT=on  RndMeth=Zero  SaturateOnIntegerOverflow=on
  Math Function{,1..3} (4 alike) : Math  Operator=square
  Product{,1..4,6..7} (7 alike) : Product  InputSameDT=on  RndMeth=Zero  SaturateOnIntegerOverflow=on
  Relational Operator : RelationalOperator  OutDataTypeStr=boolean
  Relational Operator1 : RelationalOperator  OutDataTypeStr=boolean
  Sqrt : Sqrt
  Switch1 : Switch  Criteria=u2 ~= 0  InputSameDT=off
  Switch2 : Switch  Criteria=u2 ~= 0  InputSameDT=off
  single{,1..3} (4 alike) : Constant  OutDataTypeStr=single
      settings: AttributesFormatString=%<OutDataTypeStr>
  single4 : Constant  Value=2  OutDataTypeStr=single
      settings: AttributesFormatString=%<OutDataTypeStr>
  single5 : Constant  Value=2  OutDataTypeStr=single
      settings: AttributesFormatString=%<OutDataTypeStr>
  tan : ITKLib_V14/BasicOperators/tan
  VfVDM_WhlLgtdF_N : Outport
  VfVDM_WhlLatF_N : Outport  Port=2
  wires:
  single1/1 -> Switch2/1
  Product3/1 -> Product4/1
  single5/1 -> Add3/2
  Switch2/1 -> Divide/1
  Product7/1 -> VfVDM_WhlLatF_N/1
  Product6/1 -> Product7/2
  Math Function1/1 -> Product/1
  single2/1 -> Relational Operator1/2
  single4/1 -> Divide1/4
  Add2/1 -> Divide/2
  Relational Operator/1 -> Switch1/2
  Add/1 -> Divide1/1
  [VfVDM_WhlSlipRat_coff] -> Math Function1/1
  [VfVDM_WhlSlipRat_coff] -> Add2/2
  VfACE_WhlAdhCoff_coff/1 -> Divide1/2
  Product4/1 -> VfVDM_WhlLgtdF_N/1
  KfVDM_TireCornrgStfn_Npm/1 -> Math Function3/1, [KfVDM_TireCornrgStfn_Npm]
  VfVME_WhlVertF_N/1 -> Divide1/3
  Add1/1 -> Sqrt/1
  Sqrt/1 -> Divide1/5
  VfVDM_TireSideSlipAng_deg/1 -> tan/1
  Product2/1 -> Switch2/3
  VfDTC_WhlSlipRat_coff/1 -> Switch1/3, Relational Operator/2
  Switch1/1 -> Add/1, [VfVDM_WhlSlipRat_coff]
  Add3/1 -> Product2/2
  Product1/1 -> Add1/2
  Relational Operator1/1 -> Switch2/2
  Product/1 -> Add1/1
  [KfVDM_TireCornrgStfn_Npm] -> Product6/1
  Math Function/1 -> Product/2
  Math Function2/1 -> Product1/1
  tan/1 -> Math Function2/1, [VfVDM_TanLMTireSideSlipAng_coff]
  [VfVDM_WhlSlipRat_coff] -> Product3/2
  Divide1/1 -> Relational Operator1/1, Product2/1, Add3/1
  single3/1 -> Add2/1
  [KfVDM_TireLgtdStfn_Npm] -> Product3/1
  [VfVDM_TanLMTireSideSlipAng_coff] -> Product6/2
  Divide/1 -> Product4/2, Product7/1
  single/1 -> Add/2
  VfASR_WhlSlipRat_coff/1 -> Switch1/1, Relational Operator/1
  Math Function3/1 -> Product1/2
  KfVDM_TireLgtdStfn_Npm/1 -> Math Function/1, [KfVDM_TireLgtdStfn_Npm]

== system ITKLib/Special/ControlAlgorithm/RCCirtVolt ==
  note: Equation for Electrical Model
      |
      | V_{int} = I.R_0 + R_1((V_c.C_1 + I.dt) \div (R_1.C_1 + dt))
      |
      | R_0 is series ohmic resistance
      | R_1 & C_1 are first order elements
  Curr : Inport
  Vc : Inport  Port=2
  RCMdlR0_Ohm : Inport  Port=3
  RCMdlR1_Ohm : Inport  Port=4
  RCMdlCap1_F : Inport  Port=5
  dT : Inport  Port=6
  Add3 : Sum  InputSameDT=on  SaturateOnIntegerOverflow=on
  Add4 : Sum  InputSameDT=on  SaturateOnIntegerOverflow=on
  Add5 : Sum  InputSameDT=on  SaturateOnIntegerOverflow=on
  Divide4 : Product  Inputs=*/
  Product{3,5..8} (5 alike) : Product  RndMeth=Zero
  Volt : Outport  VectorParamsAs1DForOutWhenUnconnected=off
  wires:
  Product5/1 -> Add5/1
  Curr/1 -> Product8/1, [Curr]
  Product8/1 -> Add3/1
  Product3/1 -> Add4/2
  Add4/1 -> Divide4/1
  Product6/1 -> Add4/1
  [RCMdlR1_Ohm] -> Product5/1
  Add5/1 -> Divide4/2
  Divide4/1 -> Product7/1
  Product7/1 -> Add3/2
  RCMdlR0_Ohm/1 -> Product8/2
  Add3/1 -> Volt/1
  [Curr] -> Product3/2
  RCMdlCap1_F/1 -> [RCMdlCap1_F], Product6/1
  RCMdlR1_Ohm/1 -> [RCMdlR1_Ohm], Product7/2
  dT/1 -> Add5/2, Product3/1
  Vc/1 -> Product6/2
  [RCMdlCap1_F] -> Product5/2

== system ITKLib/Special/ControlAlgorithm/RCCritCurr ==
  note: Equation from Electrical Model
      |
      | V_t = I.R_0 + R_1((V_c.C_1 + I.dt) \div (R_1.C_1 + dt))
      |
      | Rearranged with respect to current
      |
      | I = (V_t - ((R_1.C_1.V_c) \div (R_1.C_1 + dt))) \div (R_0 + ((R_1.dt) \div (R_1.C_1 + dt))
  ModelVTarget_V : Inport
  Vc : Inport  Port=2
  RCMdlR0_Ohm : Inport  Port=3
  RCMdlR1_Ohm : Inport  Port=4
  RCMdlCap1_F : Inport  Port=5
  dT : Inport  Port=6
  Add : Sum  InputSameDT=on  SaturateOnIntegerOverflow=on
  Add1 : Sum  InputSameDT=on  SaturateOnIntegerOverflow=on
  Add2 : Sum  InputSameDT=on  SaturateOnIntegerOverflow=on
  Divide1 : Product  Inputs=*/
  Divide3 : Product  Inputs=*/
  Product1 : Product  RndMeth=Zero
  Product2 : Product  RndMeth=Zero
  Product4 : Product  RndMeth=Zero
  Safe_Divide : Subsystem  RTWFcnName=Safe_Divide  RTWFileName=BoschITK_Mdl_Lib  mask(Safe_Divide){}
      mask help:
      | Safe Divide, prevents division by zero.
      |
      | if abs(denominator) > abs(eps) then
      |     output = numerator / denominator
      | elseif  denominator ≥ 0
      |     output = numerator / abs(eps)
      | else
      |     output = numerator / (-abs(eps))
      |
      |
      | Warning!
      | Use this block only when there is a risk for division by zero.
      |
      | Simulink Custom Model Library, created by MCC.
      settings: RTWFcnNameOpts=User specified  RTWFileNameOpts=User specified
      mask Display:
      | port_label('input', 1, 'x')
      | port_label('input', 2, '÷')
      | port_label('input', 3, 'eps')
  Subtract : Sum  Inputs=+-  InputSameDT=on  SaturateOnIntegerOverflow=on
  single : Constant  Value=0.00001  OutDataTypeStr=single  SampleTime=-1
      settings: AttributesFormatString=%<OutDataTypeStr>
  Curr : Outport  VectorParamsAs1DForOutWhenUnconnected=off
  wires:
  Product2/1 -> Divide3/1
  Divide3/1 -> Subtract/2
  RCMdlR1_Ohm/1 -> [RCMdlR1_Ohm], Product1/1
  RCMdlCap1_F/1 -> Product1/2
  Product1/1 -> Product2/2, Add/1, [RCMdlTau]
  Add/1 -> Divide3/2
  Vc/1 -> Product2/1
  ModelVTarget_V/1 -> Subtract/1
  [RCMdlR1_Ohm] -> Product4/1
  Product4/1 -> Divide1/1
  [RCMdlTau] -> Add2/1
  dT/1 -> Add/2, Add2/2, Product4/2
  Add2/1 -> Divide1/2
  Divide1/1 -> Add1/1
  RCMdlR0_Ohm/1 -> Add1/2
  Subtract/1 -> Safe_Divide/1(In)
  Add1/1 -> Safe_Divide/2(In1)
  Safe_Divide/1(Out) -> Curr/1
  single/1 -> Safe_Divide/3(eps)

== system ITKLib/Special/Diagramm Chapter/EmptySubsystem ==

== system ITKLib/Special/Document/PolarionID ==

== system ITKLib/TimeCounter/CounterRStep/Limit ==
  MX : Inport
  u : Inport  Port=2
  MN : Inport  Port=3
  MinMax : MinMax  Inputs=2  SaturateOnIntegerOverflow=on
  MinMax1 : MinMax  Function=max  Inputs=2  SaturateOnIntegerOverflow=on
  y : Outport  InitialOutput=0
  wires:
  MX/1 -> MinMax/1
  u/1 -> MinMax1/1
  MN/1 -> MinMax1/2
  MinMax1/1 -> MinMax/2
  MinMax/1 -> y/1

== system ITKLib/TimeCounter/CounterRStep/Limit1 ==
  MX : Inport
  u : Inport  Port=2
  MN : Inport  Port=3
  MinMax : MinMax  Inputs=2  SaturateOnIntegerOverflow=on
  MinMax1 : MinMax  Function=max  Inputs=2  SaturateOnIntegerOverflow=on
  y : Outport  InitialOutput=0
  wires:
  MX/1 -> MinMax/1
  u/1 -> MinMax1/1
  MN/1 -> MinMax1/2
  MinMax1/1 -> MinMax/2
  MinMax/1 -> y/1

== system ITKLib/TimeCounter/DebCnt/DebounceEnable ==
  bOutRangedOld : Inport
  bFailedOld : Inport  Port=2
  bEna : Inport  Port=3  OutDataTypeStr=boolean  PortDimensions=1
  bRst : Inport  Port=4
  bErr : Inport  Port=5
  Logical Operator : Logic  Operator=OR  OutDataTypeStr=boolean
  Logical Operator1 : Logic  OutDataTypeStr=boolean
  Logical Operator2 : Logic  Operator=NOT  Inputs=1  AllPortsSameDT=off  OutDataTypeStr=boolean
  Logical Operator3 : Logic  OutDataTypeStr=boolean
  Logical Operator4 : Logic  Inputs=1  AllPortsSameDT=off  OutDataTypeStr=boolean
  Relational Operator : RelationalOperator  Operator===  OutDataTypeStr=boolean
  bDebounceEna : Outport
  wires:
  bEna/1 -> Logical Operator3/2
  Logical Operator3/1 -> Logical Operator/1
  Logical Operator/1 -> bDebounceEna/1
  Relational Operator/1 -> Logical Operator1/2
  Logical Operator1/1 -> Logical Operator4/1
  Logical Operator2/1 -> Logical Operator3/1
  bOutRangedOld/1 -> Logical Operator1/1
  Logical Operator4/1 -> Logical Operator2/1
  bErr/1 -> Relational Operator/2
  bRst/1 -> Logical Operator/2
  bFailedOld/1 -> Relational Operator/1

== system ITKLib/TimeCounter/DebCnt/Debounce_OBD ==
  note: test run failure always causes fault detection counter to increment above 0
      | (so as not to double the fail detection time following a test complete with pass)
  note: only if the FaultDetectionCounter less than 0
  note: rising edge detection
  note: FailCtr <= errCtr <= RecoverCtr
  bErr : Inport
  bRst : Inport  Port=2
  FailThd : Inport  Port=3
  RecThd : Inport  Port=4
  IncrFail : Inport  Port=5
  DecrRec : Inport  Port=6
  Enable : EnablePort
  EdgeRising1 : $bdroot/Memory/EdgeRising  Tag=initial value = 0
  LORelay1 : Logic  Operator=OR  AllPortsSameDT=off  OutDataTypeStr=boolean
  Logical Operator : Logic  OutDataTypeStr=boolean
  ROLoLim : RelationalOperator  Operator=<  OutDataTypeStr=boolean  InputSameDT=off
  ROUpLim : RelationalOperator  Operator=<  OutDataTypeStr=boolean  InputSameDT=off
  RSLatch1 : $bdroot/Memory/RSLatch
  Relational Operator : RelationalOperator  Operator=<  OutDataTypeStr=boolean
  Saturation2 : Saturate  UpperLimit=int16(32766)  LowerLimit=int16(-32767)
      settings: AttributesFormatString=|
      | UpperLimit = %<UpperLimit>
      | LowLimit = %<LowerLimit>
  Sum1 : Sum  InputSameDT=on  OutDataTypeStr=int16  SaturateOnIntegerOverflow=on
  Sum2 : Sum  InputSameDT=on  OutDataTypeStr=int16  SaturateOnIntegerOverflow=on
  Switch{,2..4} (4 alike) : Switch  Criteria=u2 ~= 0  SaturateOnIntegerOverflow=off  InputSameDT=off
      settings: AttributesFormatString=Criteria : %<Criteria>
  Unit Delay : UnitDelay  SampleTime=-1  HasFrameUpgradeWarning=on
      settings: AttributesFormatString=<initial=%<x0>>
  int1 : Constant  Value=0  OutDataTypeStr=int16
      settings: AttributesFormatString=%<OutDataTypeStr>
  int16 : Constant  Value=0  OutDataTypeStr=int16
      settings: AttributesFormatString=%<OutDataTypeStr>
  bOutRanged : Outport  InitialOutput=0
  bFaild : Outport  Port=2  InitialOutput=0
  wires:
  [bRst] -> Switch2/2
  Switch2/1 -> Sum2/2, Switch3/1, Sum1/2
  Switch/1 -> Switch2/3
  int16/1 -> Switch2/1, Switch/1
  RSLatch1/1 -> bFaild/1
  Sum1/1 -> Switch4/1
  bErr/1 -> EdgeRising1/1, Switch4/2
  Logical Operator/1 -> Switch/2
  Relational Operator/1 -> Logical Operator/2
  int1/1 -> Relational Operator/2
  EdgeRising1/1 -> Logical Operator/1
  Switch3/1 -> Unit Delay/1
  bRst/1 -> [bRst], LORelay1/2
  RecThd/1 -> ROLoLim/2
  ROUpLim/1 -> RSLatch1/1, Switch3/2, bOutRanged/1  "outRanged"
  ROLoLim/1 -> LORelay1/1
  FailThd/1 -> ROUpLim/1
  LORelay1/1 -> RSLatch1/2
  Switch4/1 -> Saturation2/1
  Unit Delay/1 -> Relational Operator/1, Switch/3
  IncrFail/1 -> Sum1/1
  DecrRec/1 -> Sum2/1
  Sum2/1 -> Switch4/3
  Saturation2/1 -> Switch3/3, ROLoLim/1, ROUpLim/2

== system ITKLib/TimeCounter/Debounce/RSLatchIV ==
  S : Inport  OutDataTypeStr=boolean
  R : Inport  Port=2  OutDataTypeStr=boolean
  IV : Inport  Port=3  OutDataTypeStr=boolean
  Logical Operator1 : Logic  Operator=NOT  AllPortsSameDT=off  OutDataTypeStr=boolean
  Logical_Operator4 : Logic  AllPortsSameDT=off  OutDataTypeStr=boolean
  Logical_Operator5 : Logic  Operator=OR  AllPortsSameDT=off  OutDataTypeStr=boolean
  Number1 : Constant  Value=0  OutDataTypeStr=boolean
      settings: AttributesFormatString=%<OutDataTypeStr>
  Switch : Switch  Criteria=u2 ~= 0  SaturateOnIntegerOverflow=off  InputSameDT=off
      settings: AttributesFormatString=Criteria : %<Criteria>
  Unit Delay : UnitDelay  SampleTime=-1  HasFrameUpgradeWarning=on
      settings: AttributesFormatString=<initial=%<x0>>
  UnitDelay2 : UnitDelay  InitialCondition=1  SampleTime=-1  HasFrameUpgradeWarning=on
      settings: AttributesFormatString=<Initial=%<x0>>
  Q : Outport  OutDataTypeStr=boolean
  wires:
  Switch/1 -> Logical_Operator5/2
  Unit Delay/1 -> Switch/3
  UnitDelay2/1 -> Switch/2
  Number1/1 -> UnitDelay2/1
  IV/1 -> Switch/1
  Logical_Operator4/1 -> Unit Delay/1, Q/1
  Logical Operator1/1 -> Logical_Operator4/1
  Logical_Operator5/1 -> Logical_Operator4/2
  R/1 -> Logical Operator1/1
  S/1 -> Logical_Operator5/1

== system ITKLib/Special/ControlAlgorithm/AdrcCtrl/CalcActDrvt ==
  DlyCnt : Inport
  dT : Inport  Port=2
  y : Inport  Port=3
  Drvt : $bdroot/BasicOperators/Drvt
  ActInpDrvt : Outport
  wires:
  DlyCnt/1 -> Drvt/2
  y/1 -> Drvt/1
  dT/1 -> Drvt/3
  Drvt/1 -> ActInpDrvt/1

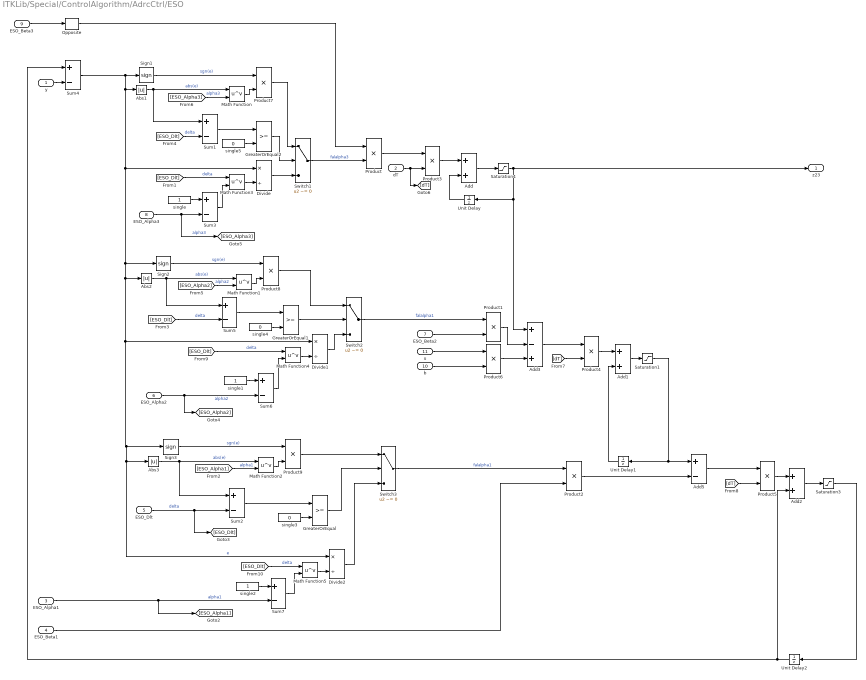
== system ITKLib/Special/ControlAlgorithm/AdrcCtrl/ESO ==
  y : Inport
  dT : Inport  Port=2
  ESO_Alpha1 : Inport  Port=3
  ESO_Beta1 : Inport  Port=4
  ESO_Dlt : Inport  Port=5
  ESO_Alpha2 : Inport  Port=6
  ESO_Beta2 : Inport  Port=7
  ESO_Alpha3 : Inport  Port=8
  ESO_Beta3 : Inport  Port=9
  b : Inport  Port=10
  u : Inport  Port=11
  Abs1 : Abs  SaturateOnIntegerOverflow=off
  Abs2 : Abs  SaturateOnIntegerOverflow=off
  Abs3 : Abs  SaturateOnIntegerOverflow=off
  Add : Sum  InputSameDT=on  SaturateOnIntegerOverflow=on
  Add1 : Sum  InputSameDT=on  SaturateOnIntegerOverflow=on
  Add2 : Sum  InputSameDT=on  SaturateOnIntegerOverflow=on
  Add3 : Sum  Inputs=+-+
  Add5 : Sum  Inputs=+-
  Divide : Product  Inputs=*/  InputSameDT=on  SaturateOnIntegerOverflow=on
  Divide1 : Product  Inputs=*/  InputSameDT=on  SaturateOnIntegerOverflow=on
  Divide2 : Product  Inputs=*/  InputSameDT=on  SaturateOnIntegerOverflow=on
  GreaterOrEqual : RelationalOperator  OutDataTypeStr=boolean
  GreaterOrEqual1 : RelationalOperator  OutDataTypeStr=boolean
  GreaterOrEqual2 : RelationalOperator  OutDataTypeStr=boolean
  Math Function{,1..5} (6 alike) : Math  Operator=pow
  Opposite : $bdroot/BasicOperators/Opposite
  Product{,1..2,6..9} (7 alike) : Product
  Product3 : Product  InputSameDT=on  SaturateOnIntegerOverflow=on
  Product4 : Product  InputSameDT=on  SaturateOnIntegerOverflow=on
  Product5 : Product  InputSameDT=on  SaturateOnIntegerOverflow=on
  Saturation1 : Saturate  UpperLimit=1000  LowerLimit=-1000
      settings: AttributesFormatString=|
      | UpperLimit = %<UpperLimit>
      | LowLimit = %<LowerLimit>
  Saturation3 : Saturate  UpperLimit=10000  LowerLimit=-10000
      settings: AttributesFormatString=|
      | UpperLimit = %<UpperLimit>
      | LowLimit = %<LowerLimit>
  Saturation4 : Saturate  UpperLimit=100  LowerLimit=-100
      settings: AttributesFormatString=|
      | UpperLimit = %<UpperLimit>
      | LowLimit = %<LowerLimit>
  Sign1 : Signum
  Sign2 : Signum
  Sign3 : Signum
  Sum{1..7} (7 alike) : Sum  Inputs=+-  SaturateOnIntegerOverflow=on
  Switch1 : Switch  Criteria=u2 ~= 0  SaturateOnIntegerOverflow=off  InputSameDT=off
  Switch2 : Switch  Criteria=u2 ~= 0  SaturateOnIntegerOverflow=off  InputSameDT=off
  Switch3 : Switch  Criteria=u2 ~= 0  SaturateOnIntegerOverflow=off  InputSameDT=off
  Unit Delay : UnitDelay  SampleTime=-1  HasFrameUpgradeWarning=on
      settings: AttributesFormatString=<initial=%<x0>>
  Unit Delay1 : UnitDelay  SampleTime=-1  HasFrameUpgradeWarning=on
      settings: AttributesFormatString=<initial=%<x0>>
  Unit Delay2 : UnitDelay  SampleTime=-1  HasFrameUpgradeWarning=on
      settings: AttributesFormatString=<initial=%<x0>>
  single : Constant  OutDataTypeStr=single  SampleTime=-1
      settings: AttributesFormatString=%<OutDataTypeStr>
  single1 : Constant  OutDataTypeStr=single  SampleTime=-1
      settings: AttributesFormatString=%<OutDataTypeStr>
  single2 : Constant  OutDataTypeStr=single  SampleTime=-1
      settings: AttributesFormatString=%<OutDataTypeStr>
  single3 : Constant  Value=0  OutDataTypeStr=single  SampleTime=-1
      settings: AttributesFormatString=%<OutDataTypeStr>
  single4 : Constant  Value=0  OutDataTypeStr=single  SampleTime=-1
      settings: AttributesFormatString=%<OutDataTypeStr>
  single5 : Constant  Value=0  OutDataTypeStr=single  SampleTime=-1
      settings: AttributesFormatString=%<OutDataTypeStr>
  z23 : Outport  VectorParamsAs1DForOutWhenUnconnected=off
  wires:
  Switch2/1 -> Product1/1  "falalpha1"
  Divide1/1 -> Switch2/3
  Product8/1 -> Switch2/1
  Sign2/1 -> Product8/1  "sgn(e)"
  Abs2/1 -> Math Function1/1, Sum5/1  "abs(e)"
  Sum5/1 -> GreaterOrEqual1/1
  [ESO_Dlt] -> Sum5/2  "delta"
  ESO_Alpha2/1 -> [ESO_Alpha2], Sum6/2  "alpha2"
  Product/1 -> Product3/1
  Abs1/1 -> Math Function/1, Sum1/1  "abs(e)"
  Switch1/1 -> Product/2  "falalpha3"
  ESO_Alpha3/1 -> [ESO_Alpha3], Sum3/2  "alpha3"
  Sign1/1 -> Product7/1  "sgn(e)"
  [ESO_Dlt] -> Sum1/2  "delta"
  Product7/1 -> Switch1/1
  Divide/1 -> Switch1/3
  Sum1/1 -> GreaterOrEqual2/1
  Opposite/1 -> Product/1
  Product1/1 -> Add3/2
  ESO_Beta2/1 -> Product1/2
  u/1 -> Product6/1
  Product6/1 -> Add3/3
  Add3/1 -> Product4/1
  Product2/1 -> Add5/2
  Add1/1 -> Saturation1/1
  ESO_Beta1/1 -> Product2/2
  Add5/1 -> Product5/1
  y/1 -> Sum4/2
  Add2/1 -> Saturation3/1
  [ESO_Alpha3] -> Math Function/2  "alpha3"
  [ESO_Alpha2] -> Math Function1/2  "alpha2"
  [ESO_Alpha1] -> Math Function2/2  "alpha1"
  Sum4/1 -> Divide2/1, Abs3/1, Sign3/1, Divide1/1, Abs2/1, Sign2/1, Divide/1, Abs1/1, Sign1/1  "e"
  ESO_Alpha1/1 -> Sum7/2, [ESO_Alpha1]  "alpha1"
  ESO_Dlt/1 -> [ESO_Dlt], Sum2/2  "delta"
  Sum2/1 -> GreaterOrEqual/1
  Abs3/1 -> Math Function2/1, Sum2/1  "abs(e)"
  Sign3/1 -> Product9/1  "sgn(e)"
  Divide2/1 -> Switch3/3
  Switch3/1 -> Product2/1  "falalpha1"
  dT/1 -> [dT], Product3/2
  Product3/1 -> Add/1
  Unit Delay/1 -> Add/2
  Product4/1 -> Add1/1
  [dT] -> Product4/2
  Unit Delay1/1 -> Add1/2
  [dT] -> Product5/2
  Product5/1 -> Add2/1
  Unit Delay2/1 -> Sum4/1, Add2/2
  Saturation4/1 -> z23/1, Unit Delay/1, Add3/1
  ESO_Beta3/1 -> Opposite/1
  b/1 -> Product6/2
  Math Function/1 -> Product7/2
  Math Function1/1 -> Product8/2
  Math Function2/1 -> Product9/2
  Product9/1 -> Switch3/1
  Sum3/1 -> Math Function3/2
  single/1 -> Sum3/1
  Math Function3/1 -> Divide/2
  Math Function4/1 -> Divide1/2
  single1/1 -> Sum6/1
  Sum6/1 -> Math Function4/2
  [ESO_Dlt] -> Math Function3/1  "delta"
  [ESO_Dlt] -> Math Function4/1  "delta"
  Sum7/1 -> Math Function5/2
  single2/1 -> Sum7/1
  Math Function5/1 -> Divide2/2
  [ESO_Dlt] -> Math Function5/1  "delta"
  GreaterOrEqual/1 -> Switch3/2
  single3/1 -> GreaterOrEqual/2
  single4/1 -> GreaterOrEqual1/2
  GreaterOrEqual1/1 -> Switch2/2
  single5/1 -> GreaterOrEqual2/2
  GreaterOrEqual2/1 -> Switch1/2
  Add/1 -> Saturation4/1
  Saturation1/1 -> Unit Delay1/1, Add5/1
  Saturation3/1 -> Unit Delay2/1
